simulink model "PIDLoop"  (R2017a)
settings: Solver=VariableStepAuto  StartTime=0.0  StopTime=10.0  RelTol=1e-3
libraries: simulink x1
settings Model: Creator=Nicoe Welch  LastModifiedBy=Nicoe Welch

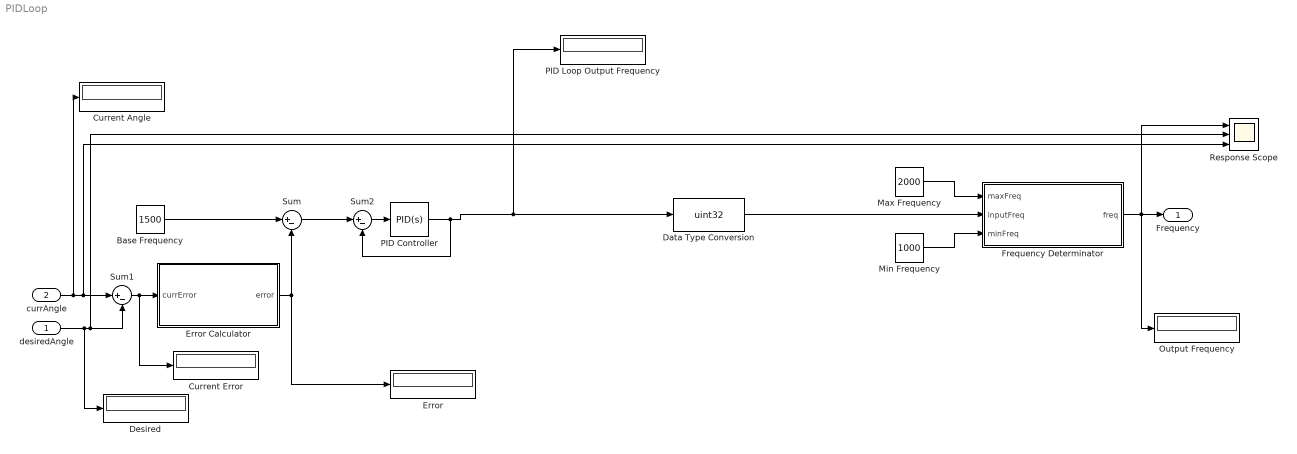
== system PIDLoop ==
  desiredAngle : Inport
  currAngle : Inport  Port=2
  Base Frequency : Constant  Value=1500
  Current Angle : Display
  Current Error : Display
  Data Type Conversion : DataTypeConversion  OutDataTypeStr=uint32  RndMeth=Nearest
  Desired : Display
  Error : Display
  Error Calculator : MATLAB Function  TreatAsAtomicUnit=on
  Frequency Determinator : MATLAB Function  TreatAsAtomicUnit=on
  Max Frequency : Constant  Value=2000  OutDataTypeStr=uint32
  Min Frequency : Constant  Value=1000  OutDataTypeStr=uint32
  Output Frequency : Display
  PID Controller : simulink/Continuous/PID Controller  Controller=PID  TimeDomain=Continuous-time  SampleTime=-1  IntegratorMethod=Forward Euler  FilterMethod=Forward Euler  Form=Parallel  UseFilter=on  ControllerParametersSource=internal  P=0  I=1  D=0  N=100  InitialConditionSource=internal  InitialConditionForIntegrator=0  InitialConditionForFilter=0  ExternalReset=none  LimitOutput=off  UpperSaturationLimit=inf  LowerSaturationLimit=-inf  LinearizeAsGain=on  AntiWindupMode=none  Kb=1  TrackingMode=off  Kt=1  PParamMin=[]  PParamMax=[]  IParamMin=[]  IParamMax=[]  DParamMin=[]  DParamMax=[]  NParamMin=[]  NParamMax=[]  KbParamMin=[]  KbParamMax=[]  KtParamMin=[]  KtParamMax=[]  POutMin=[]  POutMax=[]  IOutMin=[]  IOutMax=[]  DOutMin=[]  DOutMax=[]  NOutMin=[]  NOutMax=[]  KbOutMin=[]  KbOutMax=[]  KtOutMin=[]  KtOutMax=[]  IntegratorOutMin=[]  IntegratorOutMax=[]  FilterOutMin=[]  FilterOutMax=[]  SumOutMin=[]  SumOutMax=[]  SumI1OutMin=[]  SumI1OutMax=[]  SumI2OutMin=[]  SumI2OutMax=[]  SumI3OutMin=[]  SumI3OutMax=[]  SumDOutMin=[]  SumDOutMax=[]  SaturationOutMin=[]  SaturationOutMax=[]  IntegratorContinuousStateAttributes=''  IntegratorStateMustResolveToSignalObject=off  IntegratorRTWStateStorageClass=Auto  FilterContinuousStateAttributes=''  FilterStateMustResolveToSignalObject=off  FilterRTWStateStorageClass=Auto  DifferentiatorICPrevScaledInput=0  DifferentiatorOutMin=[]  DifferentiatorOutMax=[]  InitialConditionSetting=State (most efficient)
  PID Loop Output Frequency : Display
  Response Scope : Scope  NumInputPorts=3
  Sum : Sum  Inputs=|+-
  Sum1 : Sum  Inputs=|+-
  Sum2 : Sum  Inputs=|+-
  Frequency : Outport
  wires:
  PID Controller/1 -> Data Type Conversion/1, PID Loop Output Frequency/1, Sum2/2
  Sum/1 -> Sum2/1
  Min Frequency/1 -> Frequency Determinator/3(minFreq)
  Data Type Conversion/1 -> Frequency Determinator/2(inputFreq)
  Sum2/1 -> PID Controller/1
  Sum1/1 -> Current Error/1, Error Calculator/1(currError)
  Max Frequency/1 -> Frequency Determinator/1(maxFreq)
  Error Calculator/1(error) -> Error/1, Sum/2
  currAngle/1 -> Current Angle/1, Sum1/1, Response Scope/3
  Base Frequency/1 -> Sum/1
  desiredAngle/1 -> Desired/1, Sum1/2, Response Scope/2
  Frequency Determinator/1(freq) -> Response Scope/1, Output Frequency/1, Frequency/1

== matlab function PIDLoop/Error Calculator ==
  data: error output; currError input
function error = fcn(currError)
if currError < 40 && currError > -40
    transError = -.01080*(currError)^3 + .678*(currError)^2 + 2.124*(currError) + 22.653;
else
    if currError > 40
        transError = 500;
    else
        transError = -500;
    end
end

if currError < 0
    error = transError * -1;
elseif currError == 0
    error = currError;
else
    error = transError;
end

== matlab function PIDLoop/Frequency Determinator ==
  data: maxFreq input; inputFreq input; freq output uint32; minFreq input
function freq = fcn(maxFreq,inputFreq, minFreq)
    if( inputFreq > maxFreq ) 
        freq = maxFreq
    elseif ( inputFreq < minFreq ) 
        freq = minFreq
    else 
        freq = inputFreq
    end
